simulink library "UserBlocks"  (R2014a)
settings: Solver=ode45  SolverMode=SingleTasking  StartTime=0.0  StopTime=10.0  RelTol=1e-3
values from neighbouring files (symbols this model uses):
  a = param.a    [DSC_Control_Analysis.m]    (also in DSC_Control_Analysis_Exp.m; DSC_Speed_Control_Analysis.m; EmpiricalTireCurves.m = 1.35; FFW_Fx.m = sqrt(curvature/(2*clothoidLength)))
  b = 1.15    [EmpiricalTireCurves.m]
  Cfls = Cfl    [EC_params_nissan.m]
  Crls = Crl    [EC_params_nissan.m]
  d0 = CSTR.d0    [Ext_MPCPara.m]
  freq = Fs/2*linspace(0,1,NFFT/2)    [AACplottingcode.m]    (also in If_alpha_tp_observer.m; If_alpha_tp_observer_for_c_code.m; If_alpha_tp_observer_shoreline.m)
  Iz = param.Iz    [DSC_Control_Analysis.m]    (also in DSC_Control_Analysis_Exp.m; DSC_Speed_Control_Analysis.m; EmpiricalTireCurves.m = 1300)
  K = 10    [EC_params_nissan.m]
  Ks = -10    [EC_params_nissan.m]
  Ksl = -10    [EC_params_nissan.m]
  Kt = 40000    [EC_params_nissan.m]
  Ku = -40000    [EC_params_nissan.m]
  m = 1724    [EmpiricalTireCurves.m]
  mu_s = mu_p    (= 0.6)    [EC_params_nissan.m]    (also in EmpiricalTireCurves.m = 0.55)
  Ns = 10    [EC_params_nissan.m]
  num = num+MTnum(m)    [Build_MtMuMy.m]
  q = 1    [EC_params_nissan.m]
  Taoh = CSTR.Taoh    [Ext_MPCPara.m]
  Ts = 0.002    [DSC_Control_Analysis.m]    (also in DSC_Control_Analysis_Exp.m; DSC_Speed_Control_Analysis.m; EC_params_nissan.m; Ext_MPCPara.m = SSD.Ts)
undefined symbols (not defined in the file or in its folder): acceAmp, ack, alphaFrontSteeringLimit, alphaFrontTable, bit, c, Cfl, Crl, CSTR, dden, deltaPsiDotGain, deltDist, den, denafilt, dnum, elaDotGain, filtera, filterb, frontAlphaLookup, frontForceLookup, FuelStartCalTime, FyFtable, gpsins, h, h_roll, hal_filter_den, hal_filter_num, hwx, hwy5, initAcce, initSpeed, isDriverNoise, lkparams, mapDataFull, mapMatchingParams, maxFrontForce, maxNumSegs, mdPtrs, numafilt, param, rearAlphaLookup, rfl, rfr, rrl, rrr, sglu, SIMP, simuCond, slimFxl, slimFxu, sliml, slimMll, slimMlr, slimMul, slimMur, slimu, sr, SSD, Standard, steering_limit ... (+7)
libraries: simulink x28, slrtlib x18, UserBlocks x6, slrtsoftinglib x6, MickLibBlocks x1, DriftControllerLibrary x1
(part 6 of 6)

== matlab function UserBlocks/TTS Steering Control/Compute Steering Along Path/StaticMap/Map-Matching Primatives Dynamic Map P1/General Map-Matching Dynamic Map/mapMatchingPrimitives Dynamic Map/Embedded MATLAB Function ==
  data: e output; deltaPsi output; curvature output; isFinalSegment output; distanceToEnd output; posE input; s output; posN input; yawAngle input; enable input; mapMatchingParams input; totalSegs input; mapIsOpen input; totalMapLength input; segLength input; cumulativeLength input; EInit input; NInit input; psiInit input; kStart input; kEnd input; prevDist input; prevSeg input; seg output; currentSegmentProgress output; iterationCount output; wasMax output; deltaS output
function [e,deltaPsi,curvature,isFinalSegment,distanceToEnd,s,seg,currentSegmentProgress,iterationCount,wasMax,deltaS] = mapMatchingPrimitives(posE,posN,yawAngle,enable,mapMatchingParams,totalSegs,mapIsOpen,totalMapLength,segLength,cumulativeLength,EInit,NInit,psiInit,kStart,kEnd,prevDist,prevSeg)
% This block supports the Embedded MATLAB subset.
% See the help menu for details.

% Check to see if we're even supposed to be map matching:
if ~enable
    
    % We're not, so let's set the outputs and be done with it.
    
    %totalSegs = mapData(1,18); % The total number of segments

    e = 0;
    deltaPsi = 0;
    curvature = 0;
    isFinalSegment = 0;
    distanceToEnd = 0;
    
    s                      = max(-1,prevDist);
    seg                    = max(0,prevSeg);
    currentSegmentProgress = 0;
    iterationCount = 0;
    wasMax = 0;
    deltaS = 0;
    
    
    return;
end

%%%%%%%%%%%%%%%%%%%%%%%%%%%
% VARIABLE INITIALIZATION %
%%%%%%%%%%%%%%%%%%%%%%%%%%%

% Extract the map matching parameters that should be set in InitMapPrimitives.m
errLim                 = mapMatchingParams(1); % The maximum change in the path distance guess before considering it as having converged
fresnelIntegralErrLim  = mapMatchingParams(2); % The maximum value of a fresnel power series term before considering it as having converged
fresnelIntegralIterLim = mapMatchingParams(3); % The maximum number of iterations of the fresnel power series before deciding it won't converge
newtonRaphsonAlpha     = mapMatchingParams(4); % The scaling factor for Newton-Raphson calculation
mapMatchingIterLim     = mapMatchingParams(5); % The maximum number of iterations of the path distance guess before breaking for time concerns

% Extract the data from the mapData matrix
% segLength        = mapData(:,2); % Length of each segment
% cumulativeLength = mapData(:,3); % Total distance to the start of each segment
% EInit            = mapData(:,4); % East coordinate of start of each segment
% NInit            = mapData(:,5); % North coordinate of start of each segment
% psiInit          = mapData(:,7); % Heading of start of each segment
% kStart           = mapData(:,8); % Initial curvature of each segment
% kEnd             = mapData(:,9); % Final curvature of each segment
% 
% mapIsOpen        = mapData(1,16); % Whether the map is open (1) or closed (0)
% totalMapLength   = mapData(1,17); % The total path length of the map
% totalSegs        = mapData(1,18); % The total number of segments

% coder.varsize('segLength',[200,1]);
% % Remove extra padding
% segLength        = segLengthIn(1:totalSegs); % Length of each segment
% cumulativeLength = cumulativeLengthIn(1:totalSegs); % Total distance to the start of each segment
% EInit            = EInitIn(1:totalSegs); % East coordinate of start of each segment
% NInit            = NInitIn(1:totalSegs); % North coordinate of start of each segment
% psiInit          = psiInitIn(1:totalSegs); % Heading of start of each segment
% kStart           = kStartIn(1:totalSegs); % Initial curvature of each segment
% kEnd             = kEndIn(1:totalSegs); % Final curvature of each segment

% idx = segLengthIn ~= -1;
% segLength        = segLengthIn(idx); % Length of each segment
% cumulativeLength = cumulativeLengthIn(idx); % Total distance to the start of each segment
% EInit            = EInitIn(1:totalSegs); % East coordinate of start of each segment
% NInit            = NInitIn(1:totalSegs); % North coordinate of start of each segment
% psiInit          = psiInitIn(1:totalSegs); % Heading of start of each segment
% kStart           = kStartIn(1:totalSegs); % Initial curvature of each segment
% kEnd             = kEndIn(1:totalSegs); % Final curvature of each segment

% % Remove extra padding
% for i = 1:totalSegs
% segLength(i)        = segLengthIn(i); % Length of each segment
% cumulativeLength(i) = cumulativeLengthIn(i); % Total distance to the start of each segment
% EInit(i)            = EInitIn(i); % East coordinate of start of each segment
% NInit(i)            = NInitIn(i); % North coordinate of start of each segment
% psiInit(i)          = psiInitIn(i); % Heading of start of each segment
% kStart(i)           = kStartIn(i); % Initial curvature of each segment
% kEnd(i)             = kEndIn(i); % Final curvature of each segment
% end

% mapIsOpen        = mapData(1,16); % Whether the map is open (1) or closed (0)
% totalMapLength   = mapData(1,17); % The total path length of the map
% totalSegs        = mapData(1,18); % The total number of segments


if prevDist < 0
    
    numDisc = 100;
    
    indexSave = 1;
    distSave = 100;
    
    for j = 1:totalSegs-1
        Etest = linspace(EInit(j),EInit(j+1),numDisc)';
        Ntest = linspace(NInit(j),NInit(j+1),numDisc)';
        onesArray = linspace(1,1,numDisc)';
        
        dist = min(sqrt((posE*onesArray-Etest).^2 + (posN*onesArray-Ntest).^2));
        
        if distSave > dist
            distSave = dist;
            indexSave = j;
        end
    end
    
    
    s = cumulativeLength(indexSave);
    seg = indexSave-1;
    
else
    % Initialize the guesses based on where they were last time around
    s   = prevDist; % The total distance from the start of the map
    seg = round(prevSeg);  % The segment number of that distance
end

if s < 1
    s = 0;
    seg = 0;
end

% Initialize the variables which will control how many iterations we run
deltaS         = 2*errLim; % The change in path distance from one iteration to the next
iterationCount = 0;        % The current iteration number

% Initialize constants that will indicate whether we want sine or cosine for the conroyIntegral or fresnelPowerSeries
COS = 0;
SIN = 1;

% Initialize the other variables that will be used in calculating the output
matlabSegIndex = seg+1;
segDist = s - cumulativeLength(matlabSegIndex);
guessE = EInit(matlabSegIndex) + conroyIntegral(COS, psiInit(matlabSegIndex),kStart(matlabSegIndex),(kEnd(matlabSegIndex)-kStart(matlabSegIndex))*0.5/segLength(matlabSegIndex),0,segDist,fresnelIntegralErrLim,fresnelIntegralIterLim);
guessN = NInit(matlabSegIndex) + conroyIntegral(SIN, psiInit(matlabSegIndex),kStart(matlabSegIndex),(kEnd(matlabSegIndex)-kStart(matlabSegIndex))*0.5/segLength(matlabSegIndex),0,segDist,fresnelIntegralErrLim,fresnelIntegralIterLim);
guessPsi = psiInit(matlabSegIndex) + kStart(matlabSegIndex)*segDist + ((kEnd(matlabSegIndex)-kStart(matlabSegIndex))*0.5/segLength(matlabSegIndex))*segDist^2;
guessCurvature = kStart(matlabSegIndex) + segDist*(kEnd(matlabSegIndex)-kStart(matlabSegIndex))/segLength(matlabSegIndex);
guessEPrime = cos(guessPsi);
guessNPrime = sin(guessPsi);

% End of the variable initialization


%%%%%%%%%%%%%%%%%%
% NEWTON-RAPHSON %
%%%%%%%%%%%%%%%%%%

while(deltaS >= errLim && iterationCount < mapMatchingIterLim)
    
    % Increment the iteration count
    iterationCount = iterationCount + 1;
    
    % MATLAB indexes from 1, so we set this segement index one higher than the one we'll return
    matlabSegIndex = seg+1;
    
    % Calculate how far along the current segment we are
    segDist = s - cumulativeLength(matlabSegIndex);
    
    %%%%%%%%%%%%%%%%%%%%%%%%%%%%%%%%%%%%%%%%%%%%%%%%%%%%%%%%%%%%%%
    % Calculate various parameters associated with our new guess %
    %%%%%%%%%%%%%%%%%%%%%%%%%%%%%%%%%%%%%%%%%%%%%%%%%%%%%%%%%%%%%%
    
    % East coordinate along the path can be calculated with the Conroy Integral
    guessE = EInit(matlabSegIndex) + conroyIntegral(COS, psiInit(matlabSegIndex),kStart(matlabSegIndex),(kEnd(matlabSegIndex)-kStart(matlabSegIndex))*0.5/segLength(matlabSegIndex),0,segDist,fresnelIntegralErrLim,fresnelIntegralIterLim);
    
    % North coordinate along the path can be calculated with the Conroy Integral
    guessN = NInit(matlabSegIndex) + conroyIntegral(SIN, psiInit(matlabSegIndex),kStart(matlabSegIndex),(kEnd(matlabSegIndex)-kStart(matlabSegIndex))*0.5/segLength(matlabSegIndex),0,segDist,fresnelIntegralErrLim,fresnelIntegralIterLim);
    
    % Heading along the path = initialHeading + kStart*s + ((kEnd - kStart)/L)*s^2
    guessPsi = psiInit(matlabSegIndex) + kStart(matlabSegIndex)*segDist + ((kEnd(matlabSegIndex)-kStart(matlabSegIndex))*0.5/segLength(matlabSegIndex))*segDist^2;
    
    % Curvature scales linearly along the length of the clothoid
    guessCurvature = kStart(matlabSegIndex) + segDist*(kEnd(matlabSegIndex)-kStart(matlabSegIndex))/segLength(matlabSegIndex);
    
    % dE/ds = cos(heading)
    guessEPrime = cos(guessPsi);
    
    % dN/ds = sin(heading)
    guessNPrime = sin(guessPsi);
    
    %%%%%%%%%%%%%%%%%%%%%%%%%%%%%%%%%%%%%
    % Perform the actual Newton Raphson %
    %%%%%%%%%%%%%%%%%%%%%%%%%%%%%%%%%%%%%
    cosPsi = cos(guessPsi); % Only need to calculate cosine once...
    sinPsi = sin(guessPsi); % Only need to calculate sine once...
    
    % Evaluate the function
    err = (posN - guessN)*sinPsi + (posE - guessE)*cosPsi;
    
    % Evaluate the function's derivative
    errDeriv = -guessNPrime*sinPsi + (posN - guessN)*guessCurvature*cosPsi - guessEPrime*cosPsi - (posE - guessE)*guessCurvature*sinPsi;
    
    % Make the new guess
    newGuessDist = s - newtonRaphsonAlpha*err/errDeriv;
    
    % Record the change
    deltaS = abs(newGuessDist - s);
    
    % And now set our new guess to the variable which will carry to the next iteration
    s = newGuessDist;
    
    % Make sure our guess is on the path
    if mapIsOpen
        
        % With an open map, make sure we're not past the end of the map
        if newGuessDist >= totalMapLength
            
            % If we are, then our final guess will be the end of the map.
            % Set the guess parameters to match that position.
            s = totalMapLength - errLim;
            seg = totalSegs - 1;
            matlabSegIndex = seg+1;
            guessE = EInit(matlabSegIndex) + conroyIntegral(COS, psiInit(matlabSegIndex),kStart(matlabSegIndex),(kEnd(matlabSegIndex)-kStart(matlabSegIndex))*0.5/segLength(matlabSegIndex),0,segDist,fresnelIntegralErrLim,fresnelIntegralIterLim);
            guessN = NInit(matlabSegIndex) + conroyIntegral(SIN, psiInit(matlabSegIndex),kStart(matlabSegIndex),(kEnd(matlabSegIndex)-kStart(matlabSegIndex))*0.5/segLength(matlabSegIndex),0,segDist,fresnelIntegralErrLim,fresnelIntegralIterLim);
            guessPsi = psiInit(matlabSegIndex) + kStart(matlabSegIndex)*segDist + ((kEnd(matlabSegIndex)-kStart(matlabSegIndex))*0.5/segLength(matlabSegIndex))*segDist^2;
            guessCurvature = kStart(matlabSegIndex) + segDist*(kEnd(matlabSegIndex)-kStart(matlabSegIndex))/segLength(matlabSegIndex);
            guessEPrime = cos(guessPsi);
            guessNPrime = sin(guessPsi);
            
            break;
        end
        
        % With an open map, make sure we're not before the start
        if newGuessDist < 0
            
            % If we are, then our final guess will be the start of the map.
            % Set the guess parameters to match that position.
            s = 0;
            seg = 0;
            matlabSegIndex = seg+1;
            guessE = EInit(matlabSegIndex) + conroyIntegral(COS, psiInit(matlabSegIndex),kStart(matlabSegIndex),(kEnd(matlabSegIndex)-kStart(matlabSegIndex))*0.5/segLength(matlabSegIndex),0,segDist,fresnelIntegralErrLim,fresnelIntegralIterLim);
            guessN = NInit(matlabSegIndex) + conroyIntegral(SIN, psiInit(matlabSegIndex),kStart(matlabSegIndex),(kEnd(matlabSegIndex)-kStart(matlabSegIndex))*0.5/segLength(matlabSegIndex),0,segDist,fresnelIntegralErrLim,fresnelIntegralIterLim);
            guessPsi = psiInit(matlabSegIndex) + kStart(matlabSegIndex)*segDist + ((kEnd(matlabSegIndex)-kStart(matlabSegIndex))*0.5/segLength(matlabSegIndex))*segDist^2;
            guessCurvature = kStart(matlabSegIndex) + segDist*(kEnd(matlabSegIndex)-kStart(matlabSegIndex))/segLength(matlabSegIndex);
            guessEPrime = cos(guessPsi);
            guessNPrime = sin(guessPsi);
            
            break;
        end
    else
        % With a closed map, we just wrap around.
        
        % Subtract the total map length as necessary.
        while s >= totalMapLength
            s = s - totalMapLength;
        end
        
        % Add the total map length as necessary.
        while s < 0
            s = s + totalMapLength;
        end
            
    end
    
    % Check to see if our guess is still in the same segment
    if (s >= (cumulativeLength(matlabSegIndex)+segLength(matlabSegIndex))) || (s < cumulativeLength(matlabSegIndex))
        
        % It's not, so let's find out where it is.
        % We'll move outward our previous guess until we find it
        for i=1:(totalSegs/2 + 1)
            
            %%%%%%%%%%%%%%%%%%%%%%%%%%
            % Check the next segment %
            %%%%%%%%%%%%%%%%%%%%%%%%%%
            
            nextSeg = seg + i;
            
            % Make sure it's not before the start.
            while nextSeg < 0
                nextSeg = nextSeg + totalSegs;
            end
            
            % Make sure it's not after the end.
            while nextSeg >= totalSegs
                nextSeg = nextSeg - totalSegs;
            end
            
            matlabNextSegIndex = nextSeg + 1;
            
            % See if this guessed segment matches the distance.
            if (s >= cumulativeLength(matlabNextSegIndex)) && (s < (cumulativeLength(matlabNextSegIndex)+segLength(matlabNextSegIndex)))
                % It does, so we're done.
                seg = round(nextSeg);
                break;
            end
            
            
            %%%%%%%%%%%%%%%%%%%%%%%%%%%%%%
            % Check the previous segment %
            %%%%%%%%%%%%%%%%%%%%%%%%%%%%%%
            
            nextSeg = seg - i;
            
            % Make sure it's not before the start.
            while nextSeg < 0
                nextSeg = nextSeg + totalSegs;
            end
            
            % Make sure it's not after the end.
            while nextSeg >= totalSegs
                nextSeg = nextSeg - totalSegs;
            end
            
            matlabNextSegIndex = nextSeg + 1;
            
            % See if this guessed segment matches the distance.
            if (s >= cumulativeLength(matlabNextSegIndex)) && (s < (cumulativeLength(matlabNextSegIndex)+segLength(matlabNextSegIndex)))
                % It does, so we're done.
                seg = round(nextSeg);
                break;
            end
            
        end
        
    end
    
end

% End of the iteration scheme

%%%%%%%%%%%%%%%%%%%%%%%%%%%%%%%%%%%
% CALCULATE THE RETURN PARAMETERS %
%%%%%%%%%%%%%%%%%%%%%%%%%%%%%%%%%%%

% LATERAL ERROR is just the distance from our actual position to our guess
e = sqrt((posE - guessE)^2 + (posN - guessN)^2);

% If we're to the right of the path, switch the sign.
if ((posE-guessE)*guessNPrime-(posN-guessN)*guessEPrime)>0
    e = -e;
end

% HEADING ERROR is just the difference between the path's heading and the current heading
% This is measured counter-clockwise from the positive east axis
deltaPsi = yawAngle - guessPsi;

% Make sure it's between -pi and pi
while deltaPsi > pi
    deltaPsi = deltaPsi - 2*pi;
end
while deltaPsi < -pi
    deltaPsi = deltaPsi + 2*pi;
end

% CURVATURE was calculated earlier
curvature = guessCurvature;

% This flag just indicates whether or not we're in the final segment
if seg == (totalSegs - 1) && mapIsOpen
    isFinalSegment = 1;
else
    isFinalSegment = 0;
end

% DISTANCE TO THE END OF THE PATH is just the total path length minus our traveled distance
if mapIsOpen
    distanceToEnd = totalMapLength - s;
else
    distanceToEnd = -1;
end

% CURRENT SEGMENT PROGRESS is just our total traveled distance minus the total distance up to the start of the current segment.
matlabSegIndex = seg+1;
currentSegmentProgress = s - cumulativeLength(matlabSegIndex);
% currentSegmentProgress = max(currentSegmentProgress,0);

% matchOut = [e;deltaPsi;curvature;isFinalSegment;distanceToEnd];
% debugOut = [iterationCount;(iterationCount == mapMatchingIterLim);deltaS];
if iterationCount == mapMatchingIterLim
    wasMax = 1;
else
    wasMax = 0;
end

end

%%%%%%%%%%%%%%%%%%%%%%%%%%%%%
% END OF MAIN FUNCTION BODY %
%%%%%%%%%%%%%%%%%%%%%%%%%%%%%

%%%%%%%%%%%%%%%%%%%%
% HELPER FUNCTIONS %
%%%%%%%%%%%%%%%%%%%%

% The Conroy Intetgral evaluates integrals of the form
%       cos(a + b*x + c*x^2)dx
%              * OR *
%       sin(a + b*x + c*x^2)dx
% using the Fresnel power series
function result = conroyIntegral(trigFcn,a,b,c,lowLim,uppLim,errLim,iterLim)

    COS = 0;
    SIN = 1;

    % Make sure c is nonzero
    if abs(c) < errLim*0.0001
        if abs(b) < errLim*0.0001

            % Only a is nonzero. We're integrating a constant
            switch trigFcn
                case COS
                    result = cos(a)*(uppLim - lowLim);
                case SIN
                    result = sin(a)*(uppLim - lowLim);
                otherwise
%                     error('Unknown trigonometric function.');
            end

        else

            % We're doing ?trig(a + b*x)dx
            switch trigFcn
                case COS
                    result = sin(a + b*uppLim)/b - sin(a + b*lowLim)/b;
                case SIN
                    result = -(cos(a + b*uppLim)/b - cos(a + b*lowLim)/b);
                otherwise
%                     error('Unknown trigonometric function.');
            end
        end

        % Don't bother doing anything else
        return;

    end

    % Avoid imaginary calculations
    cIsNegative = (c < 0);
    recipSqrtC = 1/sqrt(abs(c));

    lowerFresnelLimit = (b+2*c*lowLim)*0.5*recipSqrtC;
    upperFresnelLimit = (b+2*c*uppLim)*0.5*recipSqrtC;
    trigArg = a - b^2*0.25/c;

    FresnelCosLow = fresnelPowSers(COS,0,lowerFresnelLimit,errLim,iterLim);
    FresnelSinLow = fresnelPowSers(SIN,0,lowerFresnelLimit,errLim,iterLim);
    FresnelCosUpp = fresnelPowSers(COS,0,upperFresnelLimit,errLim,iterLim);
    FresnelSinUpp = fresnelPowSers(SIN,0,upperFresnelLimit,errLim,iterLim);
    if cIsNegative
        FresnelCosLow = -1*FresnelCosLow;
        FresnelCosUpp = -1*FresnelCosUpp;
    end

    switch trigFcn

        case COS

            upperResult = recipSqrtC*(cos(trigArg)*FresnelCosUpp - sin(trigArg)*FresnelSinUpp);
            lowerResult = recipSqrtC*(cos(trigArg)*FresnelCosLow - sin(trigArg)*FresnelSinLow);
            result = upperResult - lowerResult;

        case SIN

            upperResult = recipSqrtC*(sin(trigArg)*FresnelCosUpp + cos(trigArg)*FresnelSinUpp);
            lowerResult = recipSqrtC*(sin(trigArg)*FresnelCosLow + cos(trigArg)*FresnelSinLow);
            result = upperResult - lowerResult;

        otherwise
%             error('Unknown trigonometric function.');

    end

end

% The fresnel power series
function fps = fresnelPowSers(trigFunc,lowLim,uppLim,errLim,iterLim)

    COS = 0;
    SIN = 1;

    % The type of trigonometric function determines which expansion to use
    switch trigFunc

        % The trig function is sine
        case SIN

            % Set the summation variables to zero to prepare for a summation
            fpsLow = 0;
            fpsUpp = 0;

            % Sum the lower limit until it changes less than the specified
            for i=0:iterLim-1
                nextTerm = ((-1)^(i))*(lowLim.^(i*4+3))/((i*4+3)*factorial(i*2+1));

                if abs(nextTerm) == inf || i==iterLim-1
    %                     error('The power series is not converging. Try numeric integration for such a large input.');
                elseif abs(nextTerm) > errLim
                    fpsLow = fpsLow + nextTerm;
                else
                    % we've hit the error limit
                    fpsLow = fpsLow + nextTerm;
                    break;
                end
            end

            % Sum the upper limit until it changes less than the specified
            % error limit
            for i=0:iterLim-1
                nextTerm = ((-1)^(i))*(uppLim.^(i*4+3))/((i*4+3)*factorial(i*2+1));

                if abs(nextTerm) == inf || i==iterLim-1
    %                     error('The power series is not converging. Try numeric integration for such a large input.');
                elseif abs(nextTerm) > errLim
                    fpsUpp = fpsUpp + nextTerm;
                else
                    % we've hit the error limit
                    fpsUpp = fpsUpp + nextTerm;
                    break;
                end
            end


        % The trig function is cosine
        case COS

            % Set the summation variables to zero to prepare for a summation
            fpsLow = 0;
            fpsUpp = 0;

            % Sum the given number of terms of the cos expansion solution
            for i=0:iterLim-1
                nextTerm = ((-1)^(i))*(lowLim.^(i*4+1))/((i*4+1)*factorial(i*2));

                if abs(nextTerm) == inf || i==iterLim-1
    %                     error('The power series is not converging. Try numeric integration for such a large input.');
                elseif abs(nextTerm) > errLim
                    fpsLow = fpsLow + nextTerm;
                else
                    % we've hit the error limit
                    fpsLow = fpsLow + nextTerm;
                    break;
                end
            end
            for i=0:iterLim-1
                nextTerm = ((-1)^(i))*(uppLim.^(i*4+1))/((i*4+1)*factorial(i*2));

                if abs(nextTerm) == inf || i==iterLim-1
    %                     error('The power series is not converging. Try numeric integration for such a large input.');
                elseif abs(nextTerm) > errLim
                    fpsUpp = fpsUpp + nextTerm;
                else
                    % we've hit the error limit
                    fpsUpp = fpsUpp + nextTerm;
                    break;
                end
            end

        % None of the above: the user provided an invalid trig function
        otherwise
%             error('Provided trigonometric function not valid');
    end

    % Set the output variable with the difference of these sums
    fps = fpsUpp - fpsLow;

end
